simulink model "LinearSimulation"  (R2018b)
settings: Solver=VariableStepAuto  StartTime=0.0  StopTime=10.0  RelTol=1e-3
values from neighbouring files (symbols this model uses):
  A = motor_speed_data*[1;1;-1;-1]/4    [Assignment8_bcValues.m]    (also in LinearMatrices.m = [0 0 0 0 0 0 0 -9.81 0 0 0 0;    0 0 0 0 0 0 9.81 0 0 0 0 0;; T_bc.m)
  C = PHI\Z    [Assignment8_bcValues.m]    (also in LinearMatrices.m = [0 0 0 0 0 0 0 0 0 0 0 -1;     0 0 0 0 0 0 0 0 0 0 0 0;     ; T_bc.m = phi\w)
undefined symbols (not defined in the file or in its folder): B, D
settings Model: Creator=jockabethponce  LastModifiedBy=jockabethponce

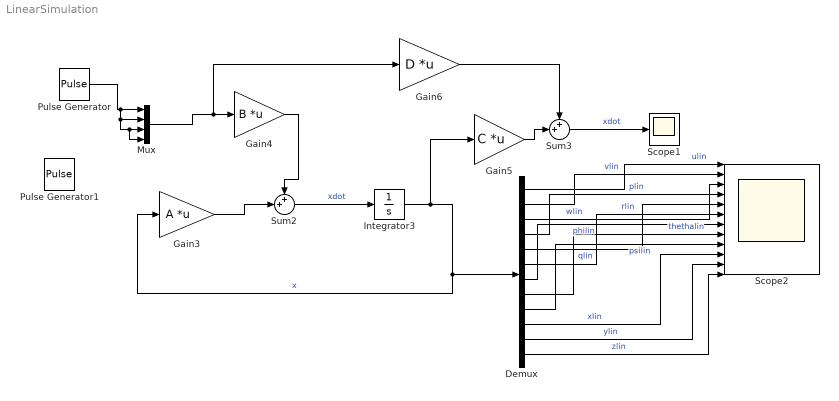
== system LinearSimulation ==
  Demux : Demux  Outputs=12
  Gain3 : Gain  Gain=A  Multiplication=Matrix(K*u) (u vector)
  Gain4 : Gain  Gain=B  Multiplication=Matrix(K*u) (u vector)
  Gain5 : Gain  Gain=C  Multiplication=Matrix(K*u) (u vector)
  Gain6 : Gain  Gain=D  Multiplication=Matrix(K*u) (u vector)
  Integrator3 : Integrator
      settings: AttributesFormatString=%<InitialCondition>
  Mux : Mux
  Pulse Generator : DiscretePulseGenerator  PulseType=Time based  Amplitude=300  Period=6  PulseWidth=4  PhaseDelay=1
  Pulse Generator1 : DiscretePulseGenerator  PulseType=Time based  Amplitude=295  Period=6  PulseWidth=4  PhaseDelay=1
  Scope1 : Scope
  Scope2 : Scope  NumInputPorts=12
  Sum2 : Sum  Inputs=++|
  Sum3 : Sum  Inputs=++|
  wires:
  Sum3/1 -> Scope1/1  "xdot"
  Integrator3/1 -> Gain5/1, Demux/1, Gain3/1  "x"
  Demux/5 -> Scope2/5  "qlin"
  Demux/8 -> Scope2/8  "thethalin"
  Demux/3 -> Scope2/3  "wlin"
  Demux/6 -> Scope2/6  "rlin"
  Demux/9 -> Scope2/9  "psilin"
  Gain3/1 -> Sum2/2
  Gain4/1 -> Sum2/1
  Demux/11 -> Scope2/11  "ylin"
  Demux/7 -> Scope2/7  "philin"
  Gain6/1 -> Sum3/1
  Sum2/1 -> Integrator3/1  "xdot"
  Gain5/1 -> Sum3/2
  Demux/4 -> Scope2/4  "plin"
  Demux/10 -> Scope2/10  "xlin"
  Mux/1 -> Gain6/1, Gain4/1
  Demux/12 -> Scope2/12  "zlin"
  Pulse Generator/1 -> Mux/4, Mux/3, Mux/2, Mux/1
  Demux/1 -> Scope2/1  "ulin"
  Demux/2 -> Scope2/2  "vlin"
